simulink model "uavCtrl_trim"  (R2024a)
settings: Solver=VariableStepAuto  StartTime=0.0  StopTime=10.0  RelTol=1e-3
values from neighbouring files (symbols this model uses):
  utrim = [-0.27394440066 -2.18120400277e-14 2.66036165513e-14 36.1693692171]    [data.mat]    (also in uavck_0.3ma.mat = [3.01593434862 -3.12927644793e-17 -4.76262648152e-17 0.40338)
settings Model: Creator=rzxha  LastModifiedBy=rzxha

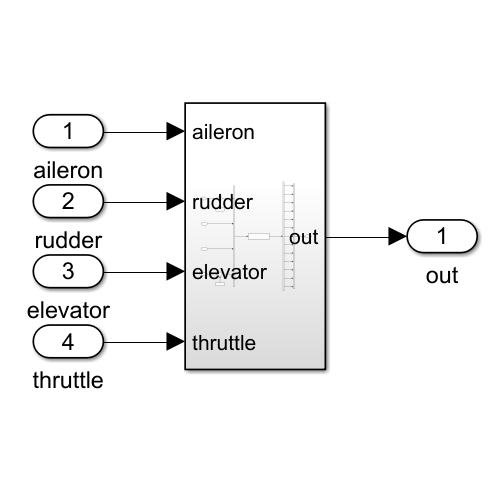
[thumbnail: Simulink's stored preview of the top-level diagram]
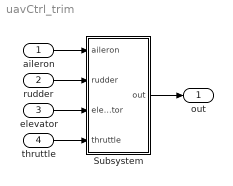
== system uavCtrl_trim ==
  aileron : Inport
  rudder : Inport  Port=2
  elevator : Inport  Port=3
  thruttle : Inport  Port=4
  Subsystem : Subsystem
  out : Outport
  wires:
  aileron/1 -> Subsystem/1(aileron)
  rudder/1 -> Subsystem/2(rudder)
  elevator/1 -> Subsystem/3(elevator)
  thruttle/1 -> Subsystem/4(thruttle)
  Subsystem/1(out) -> out/1

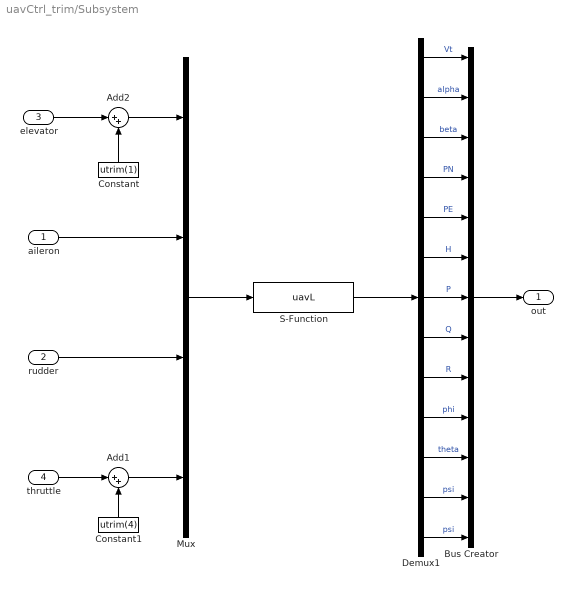
== system uavCtrl_trim/Subsystem ==
  aileron : Inport
  rudder : Inport  Port=2
  elevator : Inport  Port=3
  thruttle : Inport  Port=4
  Add1 : Sum  Inputs=|++
  Add2 : Sum  Inputs=|++
  Bus Creator : BusCreator  Inputs=13
  Constant : Constant  Value=utrim(1)
  Constant1 : Constant  Value=utrim(4)
  Demux1 : Demux  Outputs=13
  Mux : Mux
  S-Function : S-Function  FunctionName=uavL  SFunctionDeploymentMode=off  EnableBusSupport=off
  out : Outport
  wires:
  Add1/1 -> Mux/4
  thruttle/1 -> Add1/1
  Constant1/1 -> Add1/2
  rudder/1 -> Mux/3
  Demux1/4 -> Bus Creator/4  "PN"
  Add2/1 -> Mux/1
  Mux/1 -> S-Function/1
  Constant/1 -> Add2/2
  aileron/1 -> Mux/2
  elevator/1 -> Add2/1
  Demux1/11 -> Bus Creator/11  "theta"
  S-Function/1 -> Demux1/1
  Demux1/12 -> Bus Creator/12  "psi"
  Demux1/5 -> Bus Creator/5  "PE"
  Demux1/10 -> Bus Creator/10  "phi"
  Demux1/6 -> Bus Creator/6  "H"
  Demux1/2 -> Bus Creator/2  "alpha"
  Demux1/1 -> Bus Creator/1  "Vt"
  Demux1/3 -> Bus Creator/3  "beta"
  Demux1/13 -> Bus Creator/13  "psi"
  Demux1/9 -> Bus Creator/9  "R"
  Demux1/8 -> Bus Creator/8  "Q"
  Demux1/7 -> Bus Creator/7  "P"
  Bus Creator/1 -> out/1
